simulink model "gm_nrhdlSignalDetection"  (R2023b)
settings: Solver=FixedStepDiscrete  StartTime=0.0  StopTime=sl_in.stopTime  RelTol=1e-3
undefined symbols (not defined in the file or in its folder): sl_in
libraries: hdlmdlgenlib x9, hdlsllib x5, simulink x4, dsphdlfiltering2 x4, dspsrcs4 x3, whdlmod x1
(part 2 of 2)

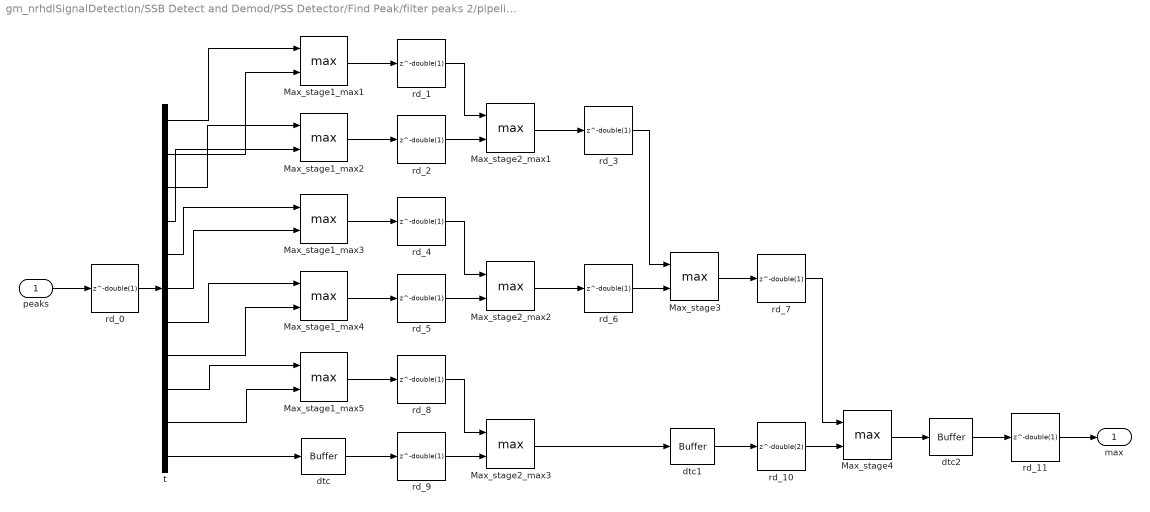
== system gm_nrhdlSignalDetection/SSB Detect and Demod/PSS Detector/Find Peak/filter peaks 2/pipelinedMax ==
  peaks : Inport  OutDataTypeStr=fixdt(1, 36, 26)  PortDimensions=[11]  SampleTime=1.62760416666667e-08
  Max_stage1_max{1..5} (5 alike) : MinMax  Function=max  Inputs=2
  Max_stage2_max1 : MinMax  Function=max  Inputs=2
  Max_stage2_max2 : MinMax  Function=max  Inputs=2
  Max_stage2_max3 : MinMax  Function=max  Inputs=2
  Max_stage3 : MinMax  Function=max  Inputs=2
  Max_stage4 : MinMax  Function=max  Inputs=2
  dtc : hdlmdlgenlib/Buffer
  dtc1 : hdlmdlgenlib/Buffer
  dtc2 : hdlmdlgenlib/Buffer
  rd_{0..9,11} (11 alike) : Delay  DelayLength=double(1)  InitialCondition=0  SampleTime=1.62760416666667e-08
  rd_10 : Delay  DelayLength=double(2)  InitialCondition=0  SampleTime=1.62760416666667e-08
  t : Demux  Outputs=11
  max : Outport  SampleTime=1.62760416666667e-08
  wires:
  peaks/1 -> rd_0/1
  t/3 -> Max_stage1_max2/1
  rd_0/1 -> t/1
  t/1 -> Max_stage1_max1/1
  t/2 -> Max_stage1_max1/2
  Max_stage2_max2/1 -> rd_6/1
  t/4 -> Max_stage1_max2/2
  t/5 -> Max_stage1_max3/1
  t/7 -> Max_stage1_max4/1
  t/6 -> Max_stage1_max3/2
  t/8 -> Max_stage1_max4/2
  t/11 -> dtc/1
  t/10 -> Max_stage1_max5/2
  t/9 -> Max_stage1_max5/1
  Max_stage1_max1/1 -> rd_1/1
  Max_stage1_max2/1 -> rd_2/1
  rd_6/1 -> Max_stage3/2
  Max_stage1_max3/1 -> rd_4/1
  Max_stage1_max4/1 -> rd_5/1
  Max_stage1_max5/1 -> rd_8/1
  dtc/1 -> rd_9/1
  rd_1/1 -> Max_stage2_max1/1
  rd_2/1 -> Max_stage2_max1/2
  rd_4/1 -> Max_stage2_max2/1
  rd_5/1 -> Max_stage2_max2/2
  rd_8/1 -> Max_stage2_max3/1
  rd_9/1 -> Max_stage2_max3/2
  Max_stage2_max1/1 -> rd_3/1
  Max_stage2_max3/1 -> dtc1/1
  rd_3/1 -> Max_stage3/1
  Max_stage3/1 -> rd_7/1
  dtc1/1 -> rd_10/1
  rd_7/1 -> Max_stage4/1
  rd_10/1 -> Max_stage4/2
  Max_stage4/1 -> dtc2/1
  dtc2/1 -> rd_11/1
  rd_11/1 -> max/1

== system gm_nrhdlSignalDetection/SSB Detect and Demod/PSS Detector/Find Peak/filter peaks 0/Delay Enabled Synchronous/Synchronous Delay ==
  u : Inport  OutDataTypeStr=fixdt(0, 32, 24)  PortDimensions=1  SampleTime=1.62760416666667e-08
  E : Inport  Port=2  OutDataTypeStr=boolean  PortDimensions=1  SampleTime=1.62760416666667e-08
  Delay : Delay  DelayLength=DelayLength  InitialCondition=InitialCondition  ShowEnablePort=on
      settings: InputPortMap=u0,e6
  StateControl : StateControl  StateControl=Synchronous
  y : Outport  SampleTime=1.62760416666667e-08
  wires:
  Delay/1 -> y/1
  u/1 -> Delay/1
  E/1 -> Delay/2

== system gm_nrhdlSignalDetection/SSB Detect and Demod/PSS Detector/Find Peak/filter peaks 1/Delay Enabled Synchronous/Synchronous Delay ==
  u : Inport  OutDataTypeStr=fixdt(0, 32, 24)  PortDimensions=1  SampleTime=1.62760416666667e-08
  E : Inport  Port=2  OutDataTypeStr=boolean  PortDimensions=1  SampleTime=1.62760416666667e-08
  Delay : Delay  DelayLength=DelayLength  InitialCondition=InitialCondition  ShowEnablePort=on
      settings: InputPortMap=u0,e6
  StateControl : StateControl  StateControl=Synchronous
  y : Outport  SampleTime=1.62760416666667e-08
  wires:
  u/1 -> Delay/1
  E/1 -> Delay/2
  Delay/1 -> y/1

== system gm_nrhdlSignalDetection/SSB Detect and Demod/PSS Detector/Find Peak/filter peaks 2/Delay Enabled Synchronous/Synchronous Delay ==
  u : Inport  OutDataTypeStr=fixdt(0, 32, 24)  PortDimensions=1  SampleTime=1.62760416666667e-08
  E : Inport  Port=2  OutDataTypeStr=boolean  PortDimensions=1  SampleTime=1.62760416666667e-08
  Delay : Delay  DelayLength=DelayLength  InitialCondition=InitialCondition  ShowEnablePort=on
      settings: InputPortMap=u0,e6
  StateControl : StateControl  StateControl=Synchronous
  y : Outport  SampleTime=1.62760416666667e-08
  wires:
  u/1 -> Delay/1
  E/1 -> Delay/2
  Delay/1 -> y/1

== matlab function gm_nrhdlSignalDetection/SSB Detect and Demod/PSS Detector/Find Peak/register PSS ID/register PSS ID ==
  data: A input; selectedPSS output; B input; C input; valid output; validIn input; start input
function [selectedPSS, valid] = registerPSSID(A, B, C, validIn, start)

persistent started pss_reg pss_valid

if isempty(pss_reg)
    started = false;
    pss_reg = fi(0,0,2,0);
    pss_valid = false;
end

valid = pss_valid;
selectedPSS = pss_reg;

if start
    started(:) = 1;
    pss_valid(:) = 0;
    pss_reg(:) = 0;
end

if started
    if validIn && ~pss_valid
        if(A||B||C)
            pss_valid(:) = true;
        
            if A == 1
                pss_reg(:) = 0;
            elseif B == 1
                pss_reg(:) = 1;
            else
                pss_reg(:) = 2;
            end
        end
    end
end

== matlab function gm_nrhdlSignalDetection/SSB Detect and Demod/PSS Detector/Stream Synchronizer/MATLAB Function/MATLAB Function ==
  data: wrAddr output; wrEn output; rdAddr output; pop input; push input; validOut output; depth parameter
function [wrAddr,wrEn,rdAddr, validOut] = ofdmDataSync(pop,push,depth)
    %#codegen
    
    coder.extrinsic('warning');
    coder.extrinsic('num2str');
    
    persistent reg level;
    
    %------------------------------------------------------------------------
    % Constants
    %------------------------------------------------------------------------
    
    addrWL = nextpow2(depth);
    
    %------------------------------------------------------------------------
    % Persistent variable initialization
    %------------------------------------------------------------------------
    
    if isempty(reg)
        
        reg = struct(...
            'wrAddr',       fi(0,0,addrWL,0,hdlfimath), ...
            'rdAddr',       fi(0,0,addrWL,0,hdlfimath), ...
            'valid',        false);
        
        % For generating warnings during simulation only.
        level = int16(0);
        
    end
    
    %------------------------------------------------------------------------
    % Outputs
    %------------------------------------------------------------------------
    
    wrAddr   = reg.wrAddr;
    wrEn     = push;
    rdAddr   = reg.rdAddr;
    validOut = reg.valid;
    
    %------------------------------------------------------------------------
    % Calculate next state values
    %------------------------------------------------------------------------
    
    % Initialize next state
    next = reg;
    
    if pop
        next.rdAddr(:)  = reg.rdAddr + 1;
        level(:)        = level - 1;
        
        if level < 0
            warning('Buffer underflow: attempt to pop data out of empty buffer.');
        end
    end
    
    if push
        next.wrAddr(:)     = reg.wrAddr+1;
        level(:)      = level+1;
        
        if level > depth            
            warning(['Buffer overflow: attempt to push data into full buffer. Level = ', num2str(level), '.']);
        end
        
    end
    
    next.valid = pop; 
    
    % Update state    
    reg = next;
end

== matlab function gm_nrhdlSignalDetection/SSB Detect and Demod/Stream Synchronizer/MATLAB Function/MATLAB Function ==
  data: wrAddr output; wrEn output; rdAddr output; pop input; push input; validOut output; depth parameter
function [wrAddr,wrEn,rdAddr, validOut] = ofdmDataSync(pop,push,depth)
    %#codegen
    
    coder.extrinsic('warning');
    coder.extrinsic('num2str');
    
    persistent reg level;
    
    %------------------------------------------------------------------------
    % Constants
    %------------------------------------------------------------------------
    
    addrWL = nextpow2(depth);
    
    %------------------------------------------------------------------------
    % Persistent variable initialization
    %------------------------------------------------------------------------
    
    if isempty(reg)
        
        reg = struct(...
            'wrAddr',       fi(0,0,addrWL,0,hdlfimath), ...
            'rdAddr',       fi(0,0,addrWL,0,hdlfimath), ...
            'valid',        false);
        
        % For generating warnings during simulation only.
        level = int16(0);
        
    end
    
    %------------------------------------------------------------------------
    % Outputs
    %------------------------------------------------------------------------
    
    wrAddr   = reg.wrAddr;
    wrEn     = push;
    rdAddr   = reg.rdAddr;
    validOut = reg.valid;
    
    %------------------------------------------------------------------------
    % Calculate next state values
    %------------------------------------------------------------------------
    
    % Initialize next state
    next = reg;
    
    if pop
        next.rdAddr(:)  = reg.rdAddr + 1;
        level(:)        = level - 1;
        
        if level < 0
            warning('Buffer underflow: attempt to pop data out of empty buffer.');
        end
    end
    
    if push
        next.wrAddr(:)     = reg.wrAddr+1;
        level(:)      = level+1;
        
        if level > depth            
            warning(['Buffer overflow: attempt to push data into full buffer. Level = ', num2str(level), '.']);
        end
        
    end
    
    next.valid = pop; 
    
    % Update state    
    reg = next;
end

== matlab function gm_nrhdlSignalDetection/SSB Detect and Demod/scsSelection/Transient Removal/Transient Removal ==
  data: dataIn input; dataOut output; validIn input; validOut output; TransientLength parameter
function [dataOut, validOut] = removeTransient(dataIn, validIn, TransientLength)
%#codegen

persistent count dataOutReg validOutReg;

if isempty(count)
    count = fi(0,0,nextpow2(TransientLength+1),0,hdlfimath);
    dataOutReg = cast(0,'like',dataIn);
    validOutReg = false;
end

dataOut  = dataOutReg;
validOut = validOutReg;

if validIn && (count == TransientLength)
    dataOutReg(:) = dataIn;
    validOutReg(:) = true;
else
    dataOutReg(:) = dataOutReg;
    validOutReg(:) = false;
end

if validIn && count ~= TransientLength
    count(:) = count + 1;
end

== matlab function gm_nrhdlSignalDetection/SSB Detect and Demod/OFDM Demodulator/OFDM Demod Controller/OFDM Demod Controller ==
  data: validIn input; startIn input; validOut output; done output
function [validOut, done] = ofdmDemodController(validIn, startIn)
    
    persistent reg
    
    Nfft = 256;
    Ncp = 18;
    numOFDMSymbols = 4;
    samplesPerOFDMSymbol = Nfft + Ncp;
    ofdmCountWL = nextpow2(samplesPerOFDMSymbol*numOFDMSymbols);
    
    if isempty(reg)
        reg = struct(...
            'valid', false, ...
            'started', false,...
            'done', false,...
            'ofdmCount', fi(0,0,ofdmCountWL,0)...
            );
    end
    
    validOut = reg.valid;
    done = reg.done;
    
    next = reg;

    if reg.done
        next.done(:) = false;
    end
        
    if startIn && validIn
        next.valid(:) = 1;
        next.started(:) = 1;
        next.ofdmCount(:) = 0;
    elseif validIn && reg.started
        next.valid(:) = 1;
        if reg.ofdmCount == samplesPerOFDMSymbol*numOFDMSymbols-2
            next.started(:) = 0;
            next.ofdmCount(:) = 0;
            next.done(:) = true;
        else
            next.ofdmCount(:) = reg.ofdmCount + 1;
        end
    else
        next.valid(:) = 0;
    end
    
    reg = next;
    
end
